simulink model "motion_example3"  (Simulink 10.0)
settings: Solver=ode45  StartTime=0.0  StopTime=3  MaxStep=1e-4  RelTol=1e-6  AbsTol=1e-6  EnableMultiTasking=on
undefined symbols (not defined in the file): Ac, Acd, Adff0, Bc, Bcd, Bdff0, Cc, Ccd, Cdff0, Dc, Ddd, Ddff0, DiscIntNeverNeededParam, Ts
libraries: motion x11, simulink3 x5, cstblocks x2
settings Model: Creator=bhisma  LastModifiedBy=bhisma  ExtModeTrigMode=oneshot  ExtModeArmWhenConnect=off
settings DataIOCC: SignalLoggingSaveFormat=ModelDataLogs
settings OptimizationCC: BooleanDataType=off  LifeSpan=auto
settings DebuggingCC: SaveWithParameterizedLinksMsg=none  SignalResolutionControl=TryResolveAllWithWarning  MultiTaskDSMMsg=warning  MultiTaskCondExecSysMsg=none  SFUnexpectedBacktrackingDiag=error  SFNoUnconditionalDefaultTransitionDiag=error  SFExecutionAtInitializationDiag=warning  ArithmeticOperatorsInVariantConditions=error
settings HardwareCC: ProdBitPerPointer=64  ProdBitPerSizeT=64  ProdBitPerPtrDiffT=64  ProdLargestAtomicFloat=Float  ProdIntDivRoundTo=Zero  ProdEndianess=LittleEndian  ProdWordSize=64  ProdHWDeviceType=Intel->x86-64 (Windows64)  TargetUnknown=on
settings SFSimCC: SimUseLocalCustomCode=on  CustomCodeUndefinedFunction=FilterOut
settings RTWCC: RTWUseLocalCustomCode=on
settings CodeAppCC: StateflowObjectComments=off
settings GRTTargetCC: TargetLangStandard=C99 (ISO)
settings ConfigComp: CovMetricSettings=dwe  CovSaveCumulativeToWorkspaceVar=off  CovSaveSingleToWorkspaceVar=off

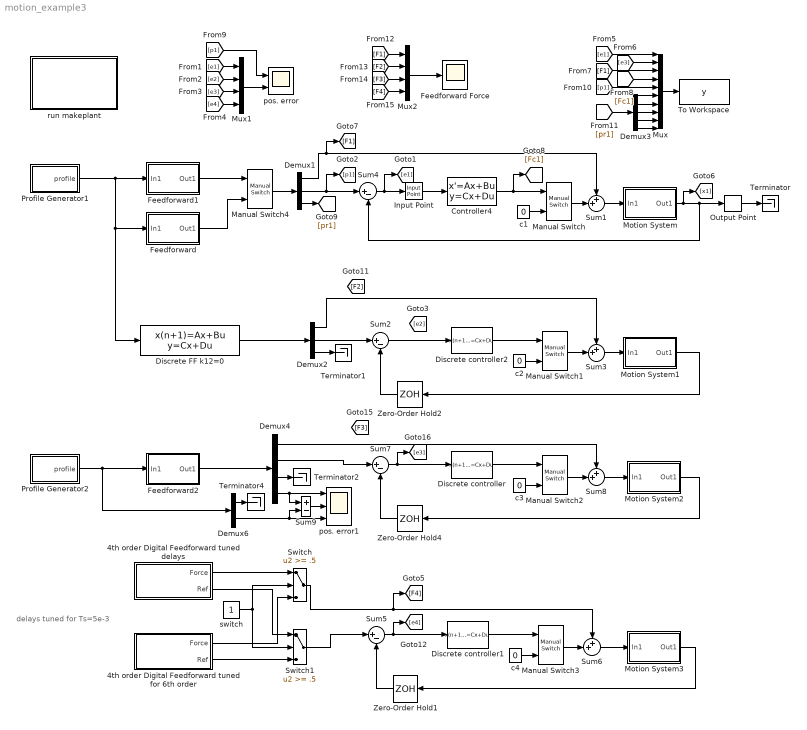
== system motion_example3 ==
  note: delays tuned for Ts=5e-3
  4th order Digital Feedforward tuned delays : Subsystem  mask{t0=.3, x=1, v=1, a=5, j=50, d=1000, Ts=Ts, r=10*eps, s=15, m1=20, m2=10, k1=10, k2=10, c=6.0e5, k12=500}
      mask prompts: t0 "Starting time:  t0 [s]"; x "Displacement:  x [m]"; v "Bound on velocity:  vmax [m/s]"; a "Bound on acceleration:  amax [m/s2]"; j "Bound on jerk: jmax [m/s3]"; d "Bound on derivative of jerk:  dmax [m/s4]"; Ts "Sampling time (0 for continuous):  Ts [s]"; r "Resolution of position [m] (default: 10*eps)"; s "Number of decimals for digitized d (default: 15)"; m1 "Actuator Mass [kg]"; m2 "Load Mass [kg]"; k1 "Actuator to ground Damping [Ns/m]"; k2 "Load to ground Damping [Ns/m]"; c "Spring Stiffness [N/m]"; k12 "Internal Damping [Ns/m]"
      mask init:
      | if length(r)==0 | length(s)==0
      | 	r=10*eps;
      | 	s=15;
      | end
      | [t,dd]=make4(abs(x),v,a,j,d,Ts,r,s);
      | t01=t0-10*eps;
      | if Ts==0
      |    [dj1,tx1,d1,j1,a1,v1,p1,tt1]=profile4(t,dd(1),.001,0);
      | else
      |    [dj1,tx1,d1,j1,a1,v1,p1,tt1]=profile4(t,dd(1),Ts/10,0);
      | end
      mask Display:
      | plot([0 dj1(1,:)+t0],[0 dj1(2,:)])
      | text(0.9*(max(dj1(1,:))+t0),0,'F\nx')
  4th order Digital Feedforward tuned for 6th order : Subsystem  mask{t0=.3, x=1, v=1, a=5, j=50, d=1000, Ts=Ts, r=10*eps, s=15, m1=20, m2=10, k1=10, k2=10, c=4.6e5, k12=500}
      mask prompts: t0 "Starting time:  t0 [s]"; x "Displacement:  x [m]"; v "Bound on velocity:  vmax [m/s]"; a "Bound on acceleration:  amax [m/s2]"; j "Bound on jerk: jmax [m/s3]"; d "Bound on derivative of jerk:  dmax [m/s4]"; Ts "Sampling time (0 for continuous):  Ts [s]"; r "Resolution of position [m] (default: 10*eps)"; s "Number of decimals for digitized d (default: 15)"; m1 "Actuator Mass [kg]"; m2 "Load Mass [kg]"; k1 "Actuator to ground Damping [Ns/m]"; k2 "Load to ground Damping [Ns/m]"; c "Spring Stiffness [N/m]"; k12 "Internal Damping [Ns/m]"
      mask init: same as motion_example3/4th order Digital Feedforward tuned delays
      mask Display:
      | plot([0 dj1(1,:)+t0],[0 dj1(2,:)])
      | text(0.9*(max(dj1(1,:))+t0),0,'F\nx')
  Controller4 : StateSpace  A=Ac  B=Bc  C=Cc  D=Dc  InitialCondition=0
  Demux1 : Demux  Outputs=[1 1 5]
  Demux2 : Demux  Outputs=[1 1 4]
  Demux3 : Demux  Outputs=5
  Demux4 : Demux  Outputs=[1 1 4 1]
  Demux6 : Demux  Outputs=2
  Discrete FF k12=0 : DiscreteStateSpace  A=Adff0  B=Bdff0  C=Cdff0  D=Ddff0  SampleTime=Ts
  Discrete controller : DiscreteStateSpace  A=Acd  B=Bcd*1.4  C=Ccd  D=Ddd  SampleTime=Ts
  Discrete controller1 : DiscreteStateSpace  A=Acd  B=Bcd*1.4  C=Ccd  D=Ddd  SampleTime=Ts
  Discrete controller2 : DiscreteStateSpace  A=Acd  B=Bcd*1.4  C=Ccd  D=Ddd  SampleTime=Ts
  Feedforward : Subsystem  BlockChoice=4th order continuous
      link override 4th order cont: k1=10  k2=10
      settings: AttributesFormatString=%<BlockChoice>  TemplateBlock=motion/Feedforward Controllers/Feedforward  MemberBlocks=2nd order continuous,2nd order discrete,3d order continuous,3d order discrete,4th order continuous,4th order digital,4th order discrete
  Feedforward Force : Scope
  Feedforward1 : Subsystem  BlockChoice=4th order continuous
      link override 4th order cont: m1=30  m2=0  k1=20  k2=0  k12=0
      settings: AttributesFormatString=%<BlockChoice>  TemplateBlock=motion/Feedforward Controllers/Feedforward  MemberBlocks=2nd order continuous,2nd order discrete,3d order continuous,3d order discrete,4th order continuous,4th order digital,4th order discrete
  Feedforward2 : Subsystem  BlockChoice=4th order digital
      link override 4th order digital: r=1e-3
      settings: AttributesFormatString=%<BlockChoice>  TemplateBlock=motion/Feedforward Controllers/Feedforward  MemberBlocks=2nd order continuous,2nd order discrete,3d order continuous,3d order discrete,4th order continuous,4th order digital,4th order discrete
  Input Point : cstblocks/Input Point
      settings: SourceProductName=Control System Toolbox  SourceProductBaseCode=CT
  Manual Switch{,1..4} (5 alike) : simulink3/Nonlinear/Manual Switch  sw=0  action=0
      settings: SourceProductName=Simulink  SourceProductBaseCode=SL
  Motion System : Subsystem  BlockChoice=Parametrized 4th order
      link override Parametrized 4th order: k1=10  k2=10  c=6e5
      settings: AttributesFormatString=%<BlockChoice>  TemplateBlock=motion/Motion Systems1/Motion System  MemberBlocks=2nd order,4th order,6th order,Parametrized 4th order
  Motion System1 : Subsystem  BlockChoice=Parametrized 4th order
      link override Parametrized 4th order: k1=10  k2=10
      settings: AttributesFormatString=%<BlockChoice>  TemplateBlock=motion/Motion Systems1/Motion System  MemberBlocks=2nd order,4th order,6th order,Parametrized 4th order
  Motion System2 : Subsystem  BlockChoice=Parametrized 4th order
      link override Parametrized 4th order: k1=10  k2=10
      settings: AttributesFormatString=%<BlockChoice>  TemplateBlock=motion/Motion Systems1/Motion System  MemberBlocks=2nd order,4th order,6th order,Parametrized 4th order
  Motion System3 : Subsystem  BlockChoice=Parametrized 4th order
      link override Parametrized 4th order: k1=10  k2=10
      settings: AttributesFormatString=%<BlockChoice>  TemplateBlock=motion/Motion Systems1/Motion System  MemberBlocks=2nd order,4th order,6th order,Parametrized 4th order
  Mux : Mux  Inputs=10
  Mux1 : Mux
  Mux2 : Mux
  Output Point : cstblocks/Output Point
      settings: SourceProductName=Control System Toolbox  SourceProductBaseCode=CT
  Profile Generator1 : Subsystem  BlockChoice=Derivative of Jerk
      link override Derivative of Jerk: Ts=Ts
      settings: AttributesFormatString=%<BlockChoice>  TemplateBlock=motion/Profile Generators/Profile Generator  MemberBlocks=Acceleration,Derivative of Jerk,Jerk,dJerk with error correction
  Profile Generator2 : Subsystem  BlockChoice=dJerk with error correction
      link override dJerk with error correction: Ts=Ts  r=1e-3  s=2
      settings: AttributesFormatString=%<BlockChoice>  TemplateBlock=motion/Profile Generators/Profile Generator  MemberBlocks=Acceleration,Derivative of Jerk,Jerk,dJerk with error correction
  Sum{1,3,6,8} (4 alike) : Sum  Inputs=++|  SaturateOnIntegerOverflow=on  InputSameDT=on  OutDataTypeStr=Inherit: Same as first input
  Sum{2,4..5,7} (4 alike) : Sum  Inputs=|+-  SaturateOnIntegerOverflow=on  InputSameDT=on  OutDataTypeStr=Inherit: Same as first input
  Sum9 : Sum  Inputs=+-  SaturateOnIntegerOverflow=on  InputSameDT=on  OutDataTypeStr=Inherit: Same as first input
  Switch : Switch  Threshold=.5  SaturateOnIntegerOverflow=on  InputSameDT=on
  Switch1 : Switch  Threshold=.5  SaturateOnIntegerOverflow=on  InputSameDT=on
  Terminator{,1..2,4} (4 alike) : Terminator
  To Workspace : ToWorkspace  VariableName=y  SaveFormat=Structure With Time  SampleTime=2e-4
  Zero-Order Hold1 : ZeroOrderHold  SampleTime=Ts
  Zero-Order Hold2 : ZeroOrderHold  SampleTime=Ts
  Zero-Order Hold4 : ZeroOrderHold  SampleTime=Ts
  c{1..4} (4 alike) : Constant  Value=0
  pos. error : Scope  NumInputPorts=2
  pos. error1 : Scope  NumInputPorts=3
  run makeplant : Subsystem  ClipboardFcn=edit makeplant
      settings: OpenFcn=makeplant  MoveFcn=edit makeplant
      mask Display: disp('MAKEPLANT\ndoubleclick to run\nmove to edit')
  switch : Constant
  wires:
  Sum1/1 -> Motion System/1(In1)
  Sum4/1 -> Input Point/1, [e1]
  Mux/1 -> To Workspace/1
  Profile Generator1/1(profile) -> Discrete FF k12=0/1, Feedforward/1(In1), Feedforward1/1(In1)
  Output Point/1 -> Terminator/1
  Motion System/1(Out1) -> Output Point/1, Sum4/2, [x1]
  Demux1/2 -> Sum4/1, [p1]
  Demux2/2 -> Sum2/1
  Discrete FF k12=0/1 -> Demux2/1
  Sum3/1 -> Motion System1/1(In1)
  Demux2/1 -> Sum3/1
  Motion System1/1(Out1) -> Zero-Order Hold2/1
  Mux1/1 -> pos. error/2
  Demux1/1 -> [F1], Sum1/1
  Mux2/1 -> Feedforward Force/1
  Demux3/1 -> Mux/6
  Demux3/2 -> Mux/7
  Demux3/3 -> Mux/8
  Demux3/4 -> Mux/9
  Sum2/1 -> Discrete controller2/1
  Demux2/3 -> Terminator1/1
  Zero-Order Hold2/1 -> Sum2/2
  [e1] -> Mux1/1
  [e2] -> Mux1/2
  [e3] -> Mux1/3
  [p1] -> pos. error/1
  [e4] -> Mux1/4
  [e1] -> Mux/1
  [e3] -> Mux/2
  [F1] -> Mux/3
  [Fc1] -> Mux/4
  [p1] -> Mux/5
  Demux1/3 -> [pr1]
  [pr1] -> Demux3/1
  Discrete controller2/1 -> Manual Switch1/1
  c1/1 -> Manual Switch/2
  Controller4/1 -> [Fc1], Manual Switch/1
  Manual Switch/1 -> Sum1/2
  c2/1 -> Manual Switch1/2
  Manual Switch1/1 -> Sum3/2
  [F1] -> Mux2/1
  [F2] -> Mux2/2
  [F3] -> Mux2/3
  [F4] -> Mux2/4
  Sum8/1 -> Motion System2/1(In1)
  Motion System2/1(Out1) -> Zero-Order Hold4/1
  Sum7/1 -> Discrete controller/1, [e3]
  Zero-Order Hold4/1 -> Sum7/2
  Discrete controller/1 -> Manual Switch2/1
  c3/1 -> Manual Switch2/2
  Manual Switch2/1 -> Sum8/2
  Sum6/1 -> Motion System3/1(In1)
  Motion System3/1(Out1) -> Zero-Order Hold1/1
  Sum5/1 -> Discrete controller1/1, [e4]
  Zero-Order Hold1/1 -> Sum5/2
  Discrete controller1/1 -> Manual Switch3/1
  c4/1 -> Manual Switch3/2
  Manual Switch3/1 -> Sum6/2
  Feedforward1/1(Out1) -> Manual Switch4/1
  Manual Switch4/1 -> Demux1/1
  Feedforward/1(Out1) -> Manual Switch4/2
  Input Point/1 -> Controller4/1
  Profile Generator2/1(profile) -> Feedforward2/1(In1), Demux6/1
  Feedforward2/1(Out1) -> Demux4/1
  Demux4/1 -> Sum8/1
  Demux4/2 -> Sum7/1
  switch/1 -> Switch/2, Switch1/2
  4th order Digital Feedforward tuned delays/1(Force) -> Switch/1
  4th order Digital Feedforward tuned delays/2(Ref) -> Switch1/1
  4th order Digital Feedforward tuned for 6th order/1(Force) -> Switch/3
  4th order Digital Feedforward tuned for 6th order/2(Ref) -> Switch1/3
  Switch/1 -> Sum6/1, [F4]
  Switch1/1 -> Sum5/1
  Demux3/5 -> Mux/10
  Demux4/3 -> Terminator2/1
  Demux4/4 -> pos. error1/1, Sum9/1
  Demux6/1 -> Terminator4/1
  Sum9/1 -> pos. error1/2
  Demux6/2 -> Sum9/2, pos. error1/3

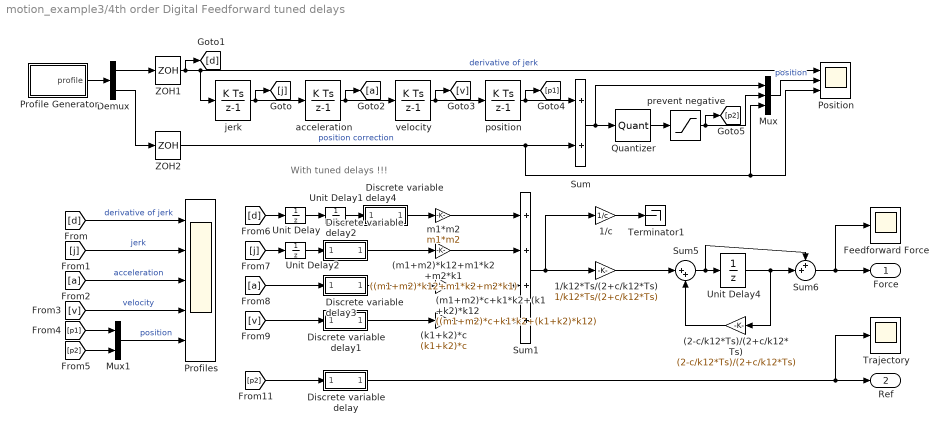
== system motion_example3/4th order Digital Feedforward tuned delays ==
  note: With tuned delays !!!
  (2-c/k12*Ts)/(2+c/k12*Ts) : Gain  Gain=(2-c/k12*Ts)/(2+c/k12*Ts)  SaturateOnIntegerOverflow=on  OutDataTypeStr=Inherit: Same as input  ParamDataTypeStr=Inherit: Same as input
  (k1+k2)*c : Gain  Gain=(k1+k2)*c  SaturateOnIntegerOverflow=on  OutDataTypeStr=Inherit: Same as input  ParamDataTypeStr=Inherit: Same as input
  (m1+m2)*c+k1*k2+(k1+k2)*k12 : Gain  Gain=((m1+m2)*c+k1*k2+(k1+k2)*k12)  SaturateOnIntegerOverflow=on  OutDataTypeStr=Inherit: Same as input  ParamDataTypeStr=Inherit: Same as input
  (m1+m2)*k12+m1*k2+m2*k1 : Gain  Gain=((m1+m2)*k12+m1*k2+m2*k1)  SaturateOnIntegerOverflow=on  OutDataTypeStr=Inherit: Same as input  ParamDataTypeStr=Inherit: Same as input
  1/c : Gain  Gain=1/c  SaturateOnIntegerOverflow=on  OutDataTypeStr=Inherit: Same as input  ParamDataTypeStr=Inherit: Same as input
  1/k12*Ts/(2+c/k12*Ts) : Gain  Gain=1/k12*Ts/(2+c/k12*Ts)  SaturateOnIntegerOverflow=on  OutDataTypeStr=Inherit: Same as input  ParamDataTypeStr=Inherit: Same as input
  Demux : Demux  Outputs=2
  Discrete variable delay : Subsystem  mask{Ts=Ts, alpha=0.5 -0.000278}
      mask prompts: Ts "Sample time"; alpha "Delay factor (between 0 and 1)"
      mask Display: disp(sprintf('%3.1f*Ts',alpha))
  Discrete variable delay1 : Subsystem  mask{Ts=Ts, alpha=0.5 -  0.000278}
      mask prompts: Ts "Sample time"; alpha "Delay factor (between 0 and 1)"
      mask Display: disp(sprintf('%3.1f*Ts',alpha))
  Discrete variable delay2 : Subsystem  mask{Ts=Ts, alpha=.50}
      mask prompts: Ts "Sample time"; alpha "Delay factor (between 0 and 1)"
      mask Display: disp(sprintf('%3.1f*Ts',alpha))
  Discrete variable delay3 : Subsystem  mask{Ts=Ts, alpha=1.00}
      mask prompts: Ts "Sample time"; alpha "Delay factor (between 0 and 1)"
      mask Display: disp(sprintf('%3.1f*Ts',alpha))
  Discrete variable delay4 : Subsystem  mask{Ts=Ts, alpha=0 + 0.095}
      mask prompts: Ts "Sample time"; alpha "Delay factor (between 0 and 1)"
      mask Display: disp(sprintf('%3.1f*Ts',alpha))
  Feedforward Force : Scope
  Mux : Mux  Inputs=3
  Mux1 : Mux  Inputs=2
  Position : Scope  NumInputPorts=3
  Profile Generator : Subsystem  BlockChoice=dJerk with error correction
      link override dJerk with error correction: t0=t0  x=x  v=v  a=a  j=j  d=d  Ts=Ts  r=r  s=s
      settings: AttributesFormatString=%<BlockChoice>  TemplateBlock=motion/Profile Generators/Profile Generator  MemberBlocks=Acceleration,Derivative of Jerk,Jerk,dJerk with error correction
  Profiles : Scope  NumInputPorts=5
  Quantizer : Quantizer  QuantizationInterval=r
  Sum : Sum  SaturateOnIntegerOverflow=on  InputSameDT=on  OutDataTypeStr=Inherit: Same as first input
  Sum1 : Sum  Inputs=++++  SaturateOnIntegerOverflow=on  InputSameDT=on  OutDataTypeStr=Inherit: Same as first input
  Sum5 : Sum  Inputs=|++  SaturateOnIntegerOverflow=on  InputSameDT=on  OutDataTypeStr=Inherit: Same as first input
  Sum6 : Sum  Inputs=++|  SaturateOnIntegerOverflow=on  InputSameDT=on  OutDataTypeStr=Inherit: Same as first input
  Terminator1 : Terminator
  Trajectory : Scope
  Unit Delay{,1..2,4} (4 alike) : UnitDelay  SampleTime=Ts
  ZOH1 : ZeroOrderHold  SampleTime=Ts
  ZOH2 : ZeroOrderHold  SampleTime=Ts
  acceleration : DiscreteIntegrator  SampleTime=Ts  ICPrevOutput=DiscIntNeverNeededParam  ICPrevScaledInput=DiscIntNeverNeededParam
  jerk : DiscreteIntegrator  SampleTime=Ts  ICPrevOutput=DiscIntNeverNeededParam  ICPrevScaledInput=DiscIntNeverNeededParam
  m1*m2 : Gain  Gain=m1*m2  SaturateOnIntegerOverflow=on  OutDataTypeStr=Inherit: Same as input  ParamDataTypeStr=Inherit: Same as input
  position : DiscreteIntegrator  SampleTime=Ts  ICPrevOutput=DiscIntNeverNeededParam  ICPrevScaledInput=DiscIntNeverNeededParam
  "prevent negative " : Saturate  UpperLimit=inf  LowerLimit=0
  velocity : DiscreteIntegrator  SampleTime=Ts  ICPrevOutput=DiscIntNeverNeededParam  ICPrevScaledInput=DiscIntNeverNeededParam
  Force : Outport
  Ref : Outport  Port=2
  wires:
  Demux/1 -> ZOH1/1
  jerk/1 -> acceleration/1, [j]
  acceleration/1 -> velocity/1, [a]
  velocity/1 -> position/1, [v]
  ZOH1/1 -> jerk/1, Position/1, [d]  "derivative of jerk"
  Demux/2 -> ZOH2/1
  Quantizer/1 -> "prevent negative "/1
  Sum/1 -> Quantizer/1, Mux/1
  Mux/1 -> Position/2  "position"
  position/1 -> Sum/1, [p1]
  ZOH2/1 -> Sum/2, Mux/3, Position/3  "position correction"
  [p1] -> Mux1/1
  [p2] -> Mux1/2
  [d] -> Profiles/1  "derivative of jerk"
  [j] -> Profiles/2  "jerk"
  [a] -> Profiles/3  "acceleration"
  [v] -> Profiles/4  "velocity"
  Mux1/1 -> Profiles/5  "position"
  [d] -> Unit Delay/1
  [j] -> Unit Delay2/1
  [a] -> Discrete variable delay3/1(In1)
  [v] -> Discrete variable delay1/1(In1)
  (m1+m2)*c+k1*k2+(k1+k2)*k12/1 -> Sum1/3
  (k1+k2)*c/1 -> Sum1/4
  Sum1/1 -> 1/c/1, 1/k12*Ts/(2+c/k12*Ts)/1
  [p2] -> Discrete variable delay/1(In1)
  Discrete variable delay/1(Out1) -> Trajectory/1, Ref/1
  "prevent negative "/1 -> Mux/2, [p2]
  Unit Delay/1 -> Unit Delay1/1
  Discrete variable delay4/1(Out1) -> m1*m2/1
  Unit Delay2/1 -> Discrete variable delay2/1(In1)
  Discrete variable delay1/1(Out1) -> (k1+k2)*c/1
  Discrete variable delay2/1(Out1) -> (m1+m2)*k12+m1*k2+m2*k1/1
  1/k12*Ts/(2+c/k12*Ts)/1 -> Sum5/1
  Sum5/1 -> Unit Delay4/1, Sum6/1
  Unit Delay4/1 -> (2-c/k12*Ts)/(2+c/k12*Ts)/1, Sum6/2
  (2-c/k12*Ts)/(2+c/k12*Ts)/1 -> Sum5/2
  Sum6/1 -> Feedforward Force/1, Force/1
  1/c/1 -> Terminator1/1
  (m1+m2)*k12+m1*k2+m2*k1/1 -> Sum1/2
  Profile Generator/1(profile) -> Demux/1
  m1*m2/1 -> Sum1/1
  Discrete variable delay3/1(Out1) -> (m1+m2)*c+k1*k2+(k1+k2)*k12/1
  Unit Delay1/1 -> Discrete variable delay4/1(In1)

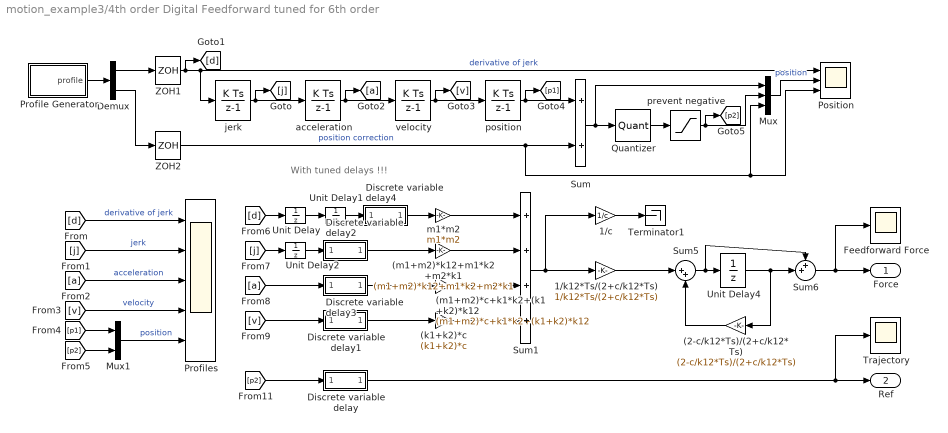
== system motion_example3/4th order Digital Feedforward tuned for 6th order ==
  note: With tuned delays !!!
  (2-c/k12*Ts)/(2+c/k12*Ts) : Gain  Gain=(2-c/k12*Ts)/(2+c/k12*Ts)  SaturateOnIntegerOverflow=on  OutDataTypeStr=Inherit: Same as input  ParamDataTypeStr=Inherit: Same as input
  (k1+k2)*c : Gain  Gain=(k1+k2)*c  SaturateOnIntegerOverflow=on  OutDataTypeStr=Inherit: Same as input  ParamDataTypeStr=Inherit: Same as input
  (m1+m2)*c+k1*k2+(k1+k2)*k12 : Gain  Gain=(m1+m2)*c+k1*k2+(k1+k2)*k12  SaturateOnIntegerOverflow=on  OutDataTypeStr=Inherit: Same as input  ParamDataTypeStr=Inherit: Same as input
  (m1+m2)*k12+m1*k2+m2*k1 : Gain  Gain=(m1+m2)*k12+m1*k2+m2*k1  SaturateOnIntegerOverflow=on  OutDataTypeStr=Inherit: Same as input  ParamDataTypeStr=Inherit: Same as input
  1/c : Gain  Gain=1/c  SaturateOnIntegerOverflow=on  OutDataTypeStr=Inherit: Same as input  ParamDataTypeStr=Inherit: Same as input
  1/k12*Ts/(2+c/k12*Ts) : Gain  Gain=1/k12*Ts/(2+c/k12*Ts)  SaturateOnIntegerOverflow=on  OutDataTypeStr=Inherit: Same as input  ParamDataTypeStr=Inherit: Same as input
  Demux : Demux  Outputs=2
  Discrete variable delay : Subsystem  mask{Ts=Ts, alpha=.4989295}
      mask prompts: Ts "Sample time"; alpha "Delay factor (between 0 and 1)"
      mask Display: disp(sprintf('%3.1f*Ts',alpha))
  Discrete variable delay1 : Subsystem  mask{Ts=Ts, alpha=.499726}
      mask prompts: Ts "Sample time"; alpha "Delay factor (between 0 and 1)"
      mask Display: disp(sprintf('%3.1f*Ts',alpha))
  Discrete variable delay2 : Subsystem  mask{Ts=Ts, alpha=.4826}
      mask prompts: Ts "Sample time"; alpha "Delay factor (between 0 and 1)"
      mask Display: disp(sprintf('%3.1f*Ts',alpha))
  Discrete variable delay3 : Subsystem  mask{Ts=Ts, alpha=1}
      mask prompts: Ts "Sample time"; alpha "Delay factor (between 0 and 1)"
      mask Display: disp(sprintf('%3.1f*Ts',alpha))
  Discrete variable delay4 : Subsystem  mask{Ts=Ts, alpha=0.03}
      mask prompts: Ts "Sample time"; alpha "Delay factor (between 0 and 1)"
      mask Display: disp(sprintf('%3.1f*Ts',alpha))
  Feedforward Force : Scope
  Mux : Mux  Inputs=3
  Mux1 : Mux  Inputs=2
  Position : Scope  NumInputPorts=3
  Profile Generator : Subsystem  BlockChoice=dJerk with error correction
      link override dJerk with error correction: t0=t0  x=x  v=v  a=a  j=j  d=d  Ts=Ts  r=r  s=s
      settings: AttributesFormatString=%<BlockChoice>  TemplateBlock=motion/Profile Generators/Profile Generator  MemberBlocks=Acceleration,Derivative of Jerk,Jerk,dJerk with error correction
  Profiles : Scope  NumInputPorts=5
  Quantizer : Quantizer  QuantizationInterval=r
  Sum : Sum  SaturateOnIntegerOverflow=on  InputSameDT=on  OutDataTypeStr=Inherit: Same as first input
  Sum1 : Sum  Inputs=++++  SaturateOnIntegerOverflow=on  InputSameDT=on  OutDataTypeStr=Inherit: Same as first input
  Sum5 : Sum  Inputs=|++  SaturateOnIntegerOverflow=on  InputSameDT=on  OutDataTypeStr=Inherit: Same as first input
  Sum6 : Sum  Inputs=++|  SaturateOnIntegerOverflow=on  InputSameDT=on  OutDataTypeStr=Inherit: Same as first input
  Terminator1 : Terminator
  Trajectory : Scope
  Unit Delay{,1..2,4} (4 alike) : UnitDelay  SampleTime=Ts
  ZOH1 : ZeroOrderHold  SampleTime=Ts
  ZOH2 : ZeroOrderHold  SampleTime=Ts
  acceleration : DiscreteIntegrator  SampleTime=Ts  ICPrevOutput=DiscIntNeverNeededParam  ICPrevScaledInput=DiscIntNeverNeededParam
  jerk : DiscreteIntegrator  SampleTime=Ts  ICPrevOutput=DiscIntNeverNeededParam  ICPrevScaledInput=DiscIntNeverNeededParam
  m1*m2 : Gain  Gain=m1*m2  SaturateOnIntegerOverflow=on  OutDataTypeStr=Inherit: Same as input  ParamDataTypeStr=Inherit: Same as input
  position : DiscreteIntegrator  SampleTime=Ts  ICPrevOutput=DiscIntNeverNeededParam  ICPrevScaledInput=DiscIntNeverNeededParam
  "prevent negative " : Saturate  UpperLimit=inf  LowerLimit=0
  velocity : DiscreteIntegrator  SampleTime=Ts  ICPrevOutput=DiscIntNeverNeededParam  ICPrevScaledInput=DiscIntNeverNeededParam
  Force : Outport
  Ref : Outport  Port=2
  wires:
  Unit Delay1/1 -> Discrete variable delay4/1(In1)
  Discrete variable delay3/1(Out1) -> (m1+m2)*c+k1*k2+(k1+k2)*k12/1
  m1*m2/1 -> Sum1/1
  Profile Generator/1(profile) -> Demux/1
  (m1+m2)*k12+m1*k2+m2*k1/1 -> Sum1/2
  1/c/1 -> Terminator1/1
  Sum6/1 -> Force/1, Feedforward Force/1
  (2-c/k12*Ts)/(2+c/k12*Ts)/1 -> Sum5/2
  Unit Delay4/1 -> Sum6/2, (2-c/k12*Ts)/(2+c/k12*Ts)/1
  Sum5/1 -> Sum6/1, Unit Delay4/1
  1/k12*Ts/(2+c/k12*Ts)/1 -> Sum5/1
  Discrete variable delay2/1(Out1) -> (m1+m2)*k12+m1*k2+m2*k1/1
  Discrete variable delay1/1(Out1) -> (k1+k2)*c/1
  Unit Delay2/1 -> Discrete variable delay2/1(In1)
  Discrete variable delay4/1(Out1) -> m1*m2/1
  Unit Delay/1 -> Unit Delay1/1
  "prevent negative "/1 -> [p2], Mux/2
  Discrete variable delay/1(Out1) -> Ref/1, Trajectory/1
  [p2] -> Discrete variable delay/1(In1)
  Sum1/1 -> 1/k12*Ts/(2+c/k12*Ts)/1, 1/c/1
  (k1+k2)*c/1 -> Sum1/4
  (m1+m2)*c+k1*k2+(k1+k2)*k12/1 -> Sum1/3
  [v] -> Discrete variable delay1/1(In1)
  [a] -> Discrete variable delay3/1(In1)
  [j] -> Unit Delay2/1
  [d] -> Unit Delay/1
  Mux1/1 -> Profiles/5  "position"
  [v] -> Profiles/4  "velocity"
  [a] -> Profiles/3  "acceleration"
  [j] -> Profiles/2  "jerk"
  [d] -> Profiles/1  "derivative of jerk"
  [p2] -> Mux1/2
  [p1] -> Mux1/1
  ZOH2/1 -> Position/3, Mux/3, Sum/2  "position correction"
  position/1 -> [p1], Sum/1
  Mux/1 -> Position/2  "position"
  Sum/1 -> Mux/1, Quantizer/1
  Quantizer/1 -> "prevent negative "/1
  Demux/2 -> ZOH2/1
  ZOH1/1 -> [d], Position/1, jerk/1  "derivative of jerk"
  velocity/1 -> [v], position/1
  acceleration/1 -> [a], velocity/1
  jerk/1 -> [j], acceleration/1
  Demux/1 -> ZOH1/1

== system motion_example3/Feedforward ==
  In1 : Inport
  4th order continuous : motion/Feedforward Controllers/4th order continuous  m1=20  m2=10  k1=10  k2=10  c=6e5  k12=500
  Out1 : Outport
  wires:
  In1/1 -> 4th order continuous/1
  4th order continuous/1 -> Out1/1

== system motion_example3/Feedforward1 ==
  In1 : Inport
  4th order continuous : motion/Feedforward Controllers/4th order continuous  m1=20  m2=10  k1=10  k2=10  c=6e5  k12=500
  Out1 : Outport
  wires:
  In1/1 -> 4th order continuous/1
  4th order continuous/1 -> Out1/1

== system motion_example3/Feedforward2 ==
  In1 : Inport
  4th order digital : motion/Feedforward Controllers/4th order digital  m1=20  m2=10  k1=10  k2=10  c=6e5  k12=500  Ts=Ts  r=1e-3
  Out1 : Outport
  wires:
  In1/1 -> 4th order digital/1
  4th order digital/1 -> Out1/1

== system motion_example3/Motion System ==
  In1 : Inport
  Parametrized 4th order : motion/Motion Systems1/Parametrized 4th order  m1=20  m2=10  k1=10  k2=10  c=6e5  k12=500
  Out1 : Outport
  wires:
  In1/1 -> Parametrized 4th order/1
  Parametrized 4th order/1 -> Out1/1

== system motion_example3/Motion System1 ==
  In1 : Inport
  Parametrized 4th order : motion/Motion Systems1/Parametrized 4th order  m1=20  m2=10  k1=10  k2=10  c=6e5  k12=500
  Out1 : Outport
  wires:
  In1/1 -> Parametrized 4th order/1
  Parametrized 4th order/1 -> Out1/1

== system motion_example3/Motion System2 ==
  In1 : Inport
  Parametrized 4th order : motion/Motion Systems1/Parametrized 4th order  m1=20  m2=10  k1=10  k2=10  c=6e5  k12=500
  Out1 : Outport
  wires:
  In1/1 -> Parametrized 4th order/1
  Parametrized 4th order/1 -> Out1/1

== system motion_example3/Motion System3 ==
  In1 : Inport
  Parametrized 4th order : motion/Motion Systems1/Parametrized 4th order  m1=20  m2=10  k1=10  k2=10  c=6e5  k12=500
  Out1 : Outport
  wires:
  In1/1 -> Parametrized 4th order/1
  Parametrized 4th order/1 -> Out1/1

== system motion_example3/Profile Generator1 ==
  Derivative of Jerk : motion/Profile Generators/Derivative of Jerk  t0=.3  x=1  v=1  a=5  j=50  d=1000  Ts=Ts
  profile : Outport
  wires:
  Derivative of Jerk/1 -> profile/1

== system motion_example3/Profile Generator2 ==
  dJerk with error correction : motion/Profile Generators/dJerk with error correction  t0=.3  x=1  v=1  a=5  j=50  d=1000  Ts=Ts  r=1e-3  s=2
  profile : Outport
  wires:
  dJerk with error correction/1 -> profile/1

== system motion_example3/run makeplant ==
  note: Run makeplant

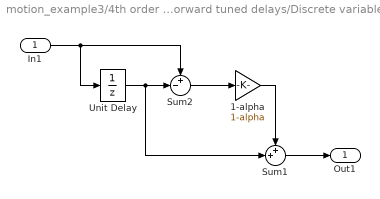
== system motion_example3/4th order Digital Feedforward tuned delays/Discrete variable delay ==
  In1 : Inport
  1-alpha : Gain  Gain=1-alpha  SaturateOnIntegerOverflow=on  OutDataTypeStr=Inherit: Same as input  ParamDataTypeStr=Inherit: Same as input
  Sum1 : Sum  Inputs=++|  SaturateOnIntegerOverflow=on  InputSameDT=on  OutDataTypeStr=Inherit: Same as first input
  Sum2 : Sum  Inputs=+-|  SaturateOnIntegerOverflow=on  InputSameDT=on  OutDataTypeStr=Inherit: Same as first input
  Unit Delay : UnitDelay  SampleTime=Ts
  Out1 : Outport
  wires:
  In1/1 -> Sum2/1, Unit Delay/1
  Unit Delay/1 -> Sum1/2, Sum2/2
  Sum1/1 -> Out1/1
  1-alpha/1 -> Sum1/1
  Sum2/1 -> 1-alpha/1

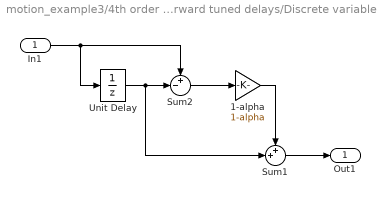
== system motion_example3/4th order Digital Feedforward tuned delays/Discrete variable delay1 ==
  In1 : Inport
  1-alpha : Gain  Gain=1-alpha  SaturateOnIntegerOverflow=on  OutDataTypeStr=Inherit: Same as input  ParamDataTypeStr=Inherit: Same as input
  Sum1 : Sum  Inputs=++|  SaturateOnIntegerOverflow=on  InputSameDT=on  OutDataTypeStr=Inherit: Same as first input
  Sum2 : Sum  Inputs=+-|  SaturateOnIntegerOverflow=on  InputSameDT=on  OutDataTypeStr=Inherit: Same as first input
  Unit Delay : UnitDelay  SampleTime=Ts
  Out1 : Outport
  wires:
  Sum2/1 -> 1-alpha/1
  1-alpha/1 -> Sum1/1
  Sum1/1 -> Out1/1
  Unit Delay/1 -> Sum2/2, Sum1/2
  In1/1 -> Unit Delay/1, Sum2/1

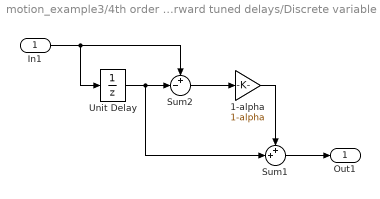
== system motion_example3/4th order Digital Feedforward tuned delays/Discrete variable delay2 ==
  In1 : Inport
  1-alpha : Gain  Gain=1-alpha  SaturateOnIntegerOverflow=on  OutDataTypeStr=Inherit: Same as input  ParamDataTypeStr=Inherit: Same as input
  Sum1 : Sum  Inputs=++|  SaturateOnIntegerOverflow=on  InputSameDT=on  OutDataTypeStr=Inherit: Same as first input
  Sum2 : Sum  Inputs=+-|  SaturateOnIntegerOverflow=on  InputSameDT=on  OutDataTypeStr=Inherit: Same as first input
  Unit Delay : UnitDelay  SampleTime=Ts
  Out1 : Outport
  wires:
  In1/1 -> Sum2/1, Unit Delay/1
  Unit Delay/1 -> Sum1/2, Sum2/2
  Sum1/1 -> Out1/1
  1-alpha/1 -> Sum1/1
  Sum2/1 -> 1-alpha/1

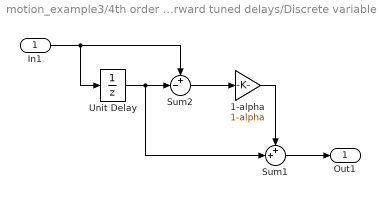
== system motion_example3/4th order Digital Feedforward tuned delays/Discrete variable delay3 ==
  In1 : Inport
  1-alpha : Gain  Gain=1-alpha  SaturateOnIntegerOverflow=on  OutDataTypeStr=Inherit: Same as input  ParamDataTypeStr=Inherit: Same as input
  Sum1 : Sum  Inputs=++|  SaturateOnIntegerOverflow=on  InputSameDT=on  OutDataTypeStr=Inherit: Same as first input
  Sum2 : Sum  Inputs=+-|  SaturateOnIntegerOverflow=on  InputSameDT=on  OutDataTypeStr=Inherit: Same as first input
  Unit Delay : UnitDelay  SampleTime=Ts
  Out1 : Outport
  wires:
  In1/1 -> Sum2/1, Unit Delay/1
  Unit Delay/1 -> Sum1/2, Sum2/2
  Sum1/1 -> Out1/1
  1-alpha/1 -> Sum1/1
  Sum2/1 -> 1-alpha/1

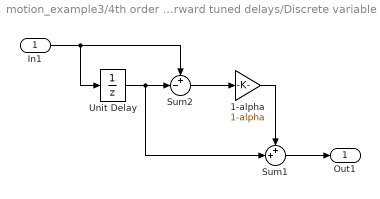
== system motion_example3/4th order Digital Feedforward tuned delays/Discrete variable delay4 ==
  In1 : Inport
  1-alpha : Gain  Gain=1-alpha  SaturateOnIntegerOverflow=on  OutDataTypeStr=Inherit: Same as input  ParamDataTypeStr=Inherit: Same as input
  Sum1 : Sum  Inputs=++|  SaturateOnIntegerOverflow=on  InputSameDT=on  OutDataTypeStr=Inherit: Same as first input
  Sum2 : Sum  Inputs=+-|  SaturateOnIntegerOverflow=on  InputSameDT=on  OutDataTypeStr=Inherit: Same as first input
  Unit Delay : UnitDelay  SampleTime=Ts
  Out1 : Outport
  wires:
  Sum2/1 -> 1-alpha/1
  1-alpha/1 -> Sum1/1
  Sum1/1 -> Out1/1
  Unit Delay/1 -> Sum2/2, Sum1/2
  In1/1 -> Unit Delay/1, Sum2/1

== system motion_example3/4th order Digital Feedforward tuned delays/Profile Generator ==
  dJerk with error correction : motion/Profile Generators/dJerk with error correction  t0=t0  x=x  v=v  a=a  j=j  d=d  Ts=Ts  r=r  s=s
  profile : Outport
  wires:
  dJerk with error correction/1 -> profile/1

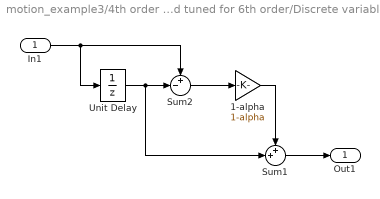
== system motion_example3/4th order Digital Feedforward tuned for 6th order/Discrete variable delay ==
  In1 : Inport
  1-alpha : Gain  Gain=1-alpha  SaturateOnIntegerOverflow=on  OutDataTypeStr=Inherit: Same as input  ParamDataTypeStr=Inherit: Same as input
  Sum1 : Sum  Inputs=++|  SaturateOnIntegerOverflow=on  InputSameDT=on  OutDataTypeStr=Inherit: Same as first input
  Sum2 : Sum  Inputs=+-|  SaturateOnIntegerOverflow=on  InputSameDT=on  OutDataTypeStr=Inherit: Same as first input
  Unit Delay : UnitDelay  SampleTime=Ts
  Out1 : Outport
  wires:
  Sum2/1 -> 1-alpha/1
  1-alpha/1 -> Sum1/1
  Sum1/1 -> Out1/1
  Unit Delay/1 -> Sum2/2, Sum1/2
  In1/1 -> Unit Delay/1, Sum2/1

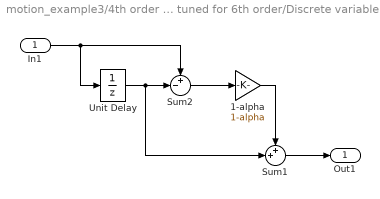
== system motion_example3/4th order Digital Feedforward tuned for 6th order/Discrete variable delay1 ==
  In1 : Inport
  1-alpha : Gain  Gain=1-alpha  SaturateOnIntegerOverflow=on  OutDataTypeStr=Inherit: Same as input  ParamDataTypeStr=Inherit: Same as input
  Sum1 : Sum  Inputs=++|  SaturateOnIntegerOverflow=on  InputSameDT=on  OutDataTypeStr=Inherit: Same as first input
  Sum2 : Sum  Inputs=+-|  SaturateOnIntegerOverflow=on  InputSameDT=on  OutDataTypeStr=Inherit: Same as first input
  Unit Delay : UnitDelay  SampleTime=Ts
  Out1 : Outport
  wires:
  In1/1 -> Sum2/1, Unit Delay/1
  Unit Delay/1 -> Sum1/2, Sum2/2
  Sum1/1 -> Out1/1
  1-alpha/1 -> Sum1/1
  Sum2/1 -> 1-alpha/1

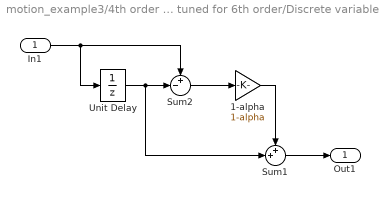
== system motion_example3/4th order Digital Feedforward tuned for 6th order/Discrete variable delay2 ==
  In1 : Inport
  1-alpha : Gain  Gain=1-alpha  SaturateOnIntegerOverflow=on  OutDataTypeStr=Inherit: Same as input  ParamDataTypeStr=Inherit: Same as input
  Sum1 : Sum  Inputs=++|  SaturateOnIntegerOverflow=on  InputSameDT=on  OutDataTypeStr=Inherit: Same as first input
  Sum2 : Sum  Inputs=+-|  SaturateOnIntegerOverflow=on  InputSameDT=on  OutDataTypeStr=Inherit: Same as first input
  Unit Delay : UnitDelay  SampleTime=Ts
  Out1 : Outport
  wires:
  Sum2/1 -> 1-alpha/1
  1-alpha/1 -> Sum1/1
  Sum1/1 -> Out1/1
  Unit Delay/1 -> Sum2/2, Sum1/2
  In1/1 -> Unit Delay/1, Sum2/1

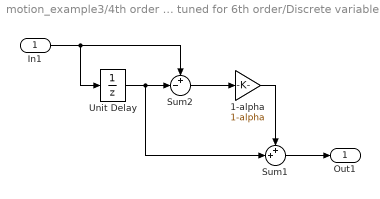
== system motion_example3/4th order Digital Feedforward tuned for 6th order/Discrete variable delay3 ==
  In1 : Inport
  1-alpha : Gain  Gain=1-alpha  SaturateOnIntegerOverflow=on  OutDataTypeStr=Inherit: Same as input  ParamDataTypeStr=Inherit: Same as input
  Sum1 : Sum  Inputs=++|  SaturateOnIntegerOverflow=on  InputSameDT=on  OutDataTypeStr=Inherit: Same as first input
  Sum2 : Sum  Inputs=+-|  SaturateOnIntegerOverflow=on  InputSameDT=on  OutDataTypeStr=Inherit: Same as first input
  Unit Delay : UnitDelay  SampleTime=Ts
  Out1 : Outport
  wires:
  Sum2/1 -> 1-alpha/1
  1-alpha/1 -> Sum1/1
  Sum1/1 -> Out1/1
  Unit Delay/1 -> Sum2/2, Sum1/2
  In1/1 -> Unit Delay/1, Sum2/1

== system motion_example3/4th order Digital Feedforward tuned for 6th order/Discrete variable delay4 ==
  In1 : Inport
  1-alpha : Gain  Gain=1-alpha  SaturateOnIntegerOverflow=on  OutDataTypeStr=Inherit: Same as input  ParamDataTypeStr=Inherit: Same as input
  Sum1 : Sum  Inputs=++|  SaturateOnIntegerOverflow=on  InputSameDT=on  OutDataTypeStr=Inherit: Same as first input
  Sum2 : Sum  Inputs=+-|  SaturateOnIntegerOverflow=on  InputSameDT=on  OutDataTypeStr=Inherit: Same as first input
  Unit Delay : UnitDelay  SampleTime=Ts
  Out1 : Outport
  wires:
  In1/1 -> Sum2/1, Unit Delay/1
  Unit Delay/1 -> Sum1/2, Sum2/2
  Sum1/1 -> Out1/1
  1-alpha/1 -> Sum1/1
  Sum2/1 -> 1-alpha/1

== system motion_example3/4th order Digital Feedforward tuned for 6th order/Profile Generator ==
  dJerk with error correction : motion/Profile Generators/dJerk with error correction  t0=t0  x=x  v=v  a=a  j=j  d=d  Ts=Ts  r=r  s=s
  profile : Outport
  wires:
  dJerk with error correction/1 -> profile/1
